simulink model "lab3"  (Simulink 7.7)
settings: Solver=ode45  StartTime=0.0  StopTime=10.0  RelTol=1e-3
libraries: cstblocks x3
settings Model: Creator=Muhammad Ali khan  LastModifiedBy=Muhammad Ali khan

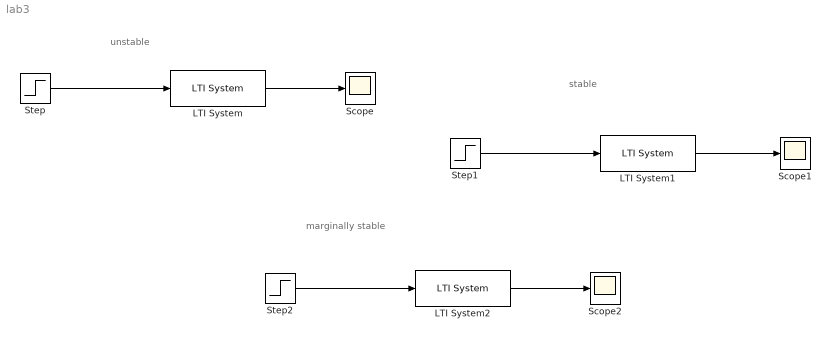
== system lab3 ==
  note: stable
  note: unstable
  note: marginally stable
  LTI System : cstblocks/LTI System  SystemSampleTime=-1  sys=tf([1 2 5],[-1 2 1])  IC=[]
  LTI System1 : cstblocks/LTI System  SystemSampleTime=-1  sys=tf([1 2 5],[5 4 2])  IC=[]
  LTI System2 : cstblocks/LTI System  SystemSampleTime=-1  sys=tf([1 2 4],[1 0 1])  IC=[]
  Scope : Scope
  Scope1 : Scope
  Scope2 : Scope
      settings: SaveName=ScopeData2
  Step : Step  SampleTime=0
  Step1 : Step  SampleTime=0
  Step2 : Step  SampleTime=0
  wires:
  Step/1 -> LTI System/1
  LTI System/1 -> Scope/1
  Step1/1 -> LTI System1/1
  LTI System1/1 -> Scope1/1
  Step2/1 -> LTI System2/1
  LTI System2/1 -> Scope2/1
